simulink model "Control_v4_desat0"  (R2020b)
settings: Solver=FixedStepAuto  StartTime=0.0  StopTime=t_sim  FixedStep=TimeStep  RelTol=1e-3
values from neighbouring files (symbols this model uses):
  date_IGRF = [date.year,date.month,date.day]    [main_SCA_v3.m]
  MODE = 2    [main_SCA_alt.m]    (also in main_SCA_v3.m)
  nmax = 2    [main_SCA.m]    (also in main_SCA_alt.m; main_SCA_v3.m)
  Use_IGRF = 0    [main_SCA.m]    (also in main_SCA_alt.m; main_SCA_v3.m)
undefined symbols (not defined in the file or in its folder): att, date, deg, DipoleMod, DiscIntNeverNeededParam, IonSataero, km, orbit, rad, s, sat
libraries: vrlib x16, aerolibconvert2 x13, aerolibutil x13, sharedtransform x11, dspmathops x10, simulink x5, sharedutil x3, simulink_extras x2, dspstat3 x1, aerolibatmos2 x1, aerolibobsolete x1, aerolibcelestial x1
(part 2 of 3)

== system Control_v4_desat0/Physical Model/Magnetorquer physics ==
  note: On pourrait aussi changer les blocs
      | magnétocoupleurs pour sortir les intensités
  Mag vector command : Inport
  B_IGRF_body (vecteur) : Inport  Port=2
  Add1 : Sum  Inputs=+++
  Cross Product : vrlib/Utilities/Cross Product
  Demux : Demux  Outputs=3
  Magnétocoupleur 1 : Subsystem
  Magnétocoupleur 2 : Subsystem
  Magnétocoupleur 3 : Subsystem
  Couple (vect) : Outport  PortDimensions=3  VectorParamsAs1DForOutWhenUnconnected=off
  Real mag moments vector : Outport  Port=2  VectorParamsAs1DForOutWhenUnconnected=off
  wires:
  Add1/1 -> Real mag moments vector/1, Cross Product/1  "M_real"
  Demux/1 -> Magnétocoupleur 1/1(m_in (scalar))
  Demux/2 -> Magnétocoupleur 2/1(m_in (scalar))
  Demux/3 -> Magnétocoupleur 3/1(m_in (scalar))
  Mag vector command/1 -> Demux/1  "m_c"
  Magnétocoupleur 2/1(m_out (vect)) -> Add1/2
  Magnétocoupleur 1/1(m_out (vect)) -> Add1/1
  Magnétocoupleur 3/1(m_out (vect)) -> Add1/3
  Cross Product/1 -> Couple (vect)/1  "T_body"
  B_IGRF_body (vecteur)/1 -> Cross Product/2

== system Control_v4_desat0/Physical Model/Thruster ==
  On/Off (Boolean) : Inport  OutDataTypeStr=boolean
  Constant : Constant  Value=0
  Cross Product : vrlib/Utilities/Cross Product
  If : If  IfExpression=u1
  If Action Subsystem : Subsystem  TreatAsAtomicUnit=on
  If Action Subsystem1 : Subsystem  TreatAsAtomicUnit=on
  Merge : Merge
  Product : Product
  Sum : Sum  Inputs=|+-
  Thruster Force : Constant  Value=sat.thruster.force
  unit vector of thrust : Constant  Value=sat.thruster.dir
  vector G-Thrust point : Constant  Value=sat.thruster.point
  vector G-Thrust point1 : Constant  Value=sat.CoG
  Force (G_sat) : Outport  VectorParamsAs1DForOutWhenUnconnected=off
  Moment (G_sat) : Outport  Port=2  VectorParamsAs1DForOutWhenUnconnected=off
  wires:
  Product/1 -> Force (G_sat)/1, Cross Product/2
  Sum/1 -> Cross Product/1
  unit vector of thrust/1 -> Product/1
  Cross Product/1 -> Moment (G_sat)/1
  Thruster Force/1 -> If Action Subsystem/1(In1)
  On/Off (Boolean)/1 -> If/1
  If/1 -> If Action Subsystem/Action
  If/2 -> If Action Subsystem1/Action
  If Action Subsystem1/1(Out1) -> Merge/2
  If Action Subsystem/1(Out1) -> Merge/1
  Merge/1 -> Product/2
  Constant/1 -> If Action Subsystem1/1(In1)
  vector G-Thrust point/1 -> Sum/1
  vector G-Thrust point1/1 -> Sum/2

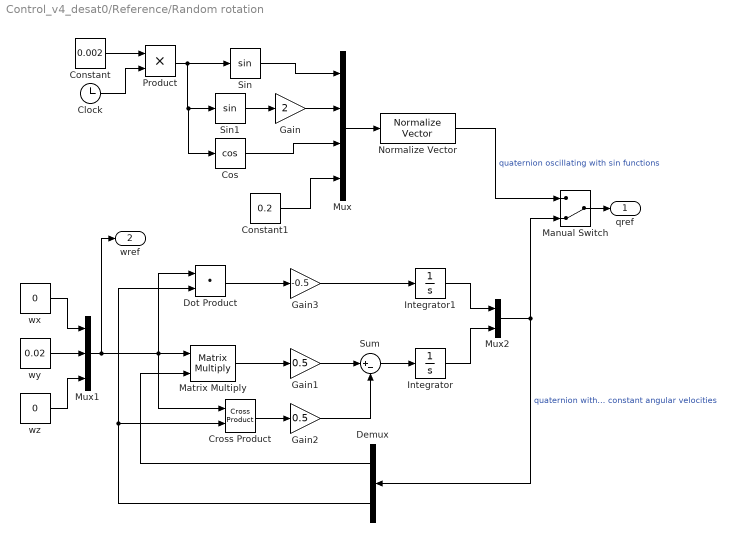
== system Control_v4_desat0/Reference/Random rotation ==
  Clock : Clock
      settings: Decimation=TimeStep
  Constant : Constant  Value=0.002
  Constant1 : Constant  Value=0.2
  Cos : Trigonometry  Operator=cos
  Cross Product : vrlib/Utilities/Cross Product
  Demux : Demux  Outputs=[1;3]
  Dot Product : DotProduct  InputSameDT=on  OutDataTypeStr=Inherit: Inherit via internal rule
  Gain : Gain  Gain=2
  Gain1 : Gain  Gain=0.5
  Gain2 : Gain  Gain=0.5
  Gain3 : Gain  Gain=-0.5
  Integrator : Integrator  InitialCondition=[0;0;0]
  Integrator1 : Integrator  InitialCondition=1
  Manual Switch : ManualSwitch  CurrentSetting=0
  Matrix Multiply : Product  Multiplication=Matrix(*)
  Mux : Mux
  Mux1 : Mux  Inputs=3
  Mux2 : Mux  Inputs=[1;3]
  Normalize Vector : vrlib/Utilities/Normalize Vector  maxzero=0
  Product : Product
  Sin : Trigonometry
  Sin1 : Trigonometry
  Sum : Sum  Inputs=|+-
  wx : Constant  Value=0
  wy : Constant  Value=0.02
  wz : Constant  Value=0
  qref : Outport
  wref : Outport  Port=2
  wires:
  Mux/1 -> Normalize Vector/1
  Normalize Vector/1 -> Manual Switch/1  "quaternion oscillating with sin functions"
  Constant/1 -> Product/1
  Clock/1 -> Product/2
  Product/1 -> Cos/1, Sin1/1, Sin/1
  Sin/1 -> Mux/1
  Sin1/1 -> Gain/1
  Gain/1 -> Mux/2
  Cos/1 -> Mux/3
  Constant1/1 -> Mux/4
  Manual Switch/1 -> qref/1
  wx/1 -> Mux1/1
  wy/1 -> Mux1/2
  wz/1 -> Mux1/3
  Mux1/1 -> wref/1, Dot Product/1, Cross Product/1, Matrix Multiply/1
  Matrix Multiply/1 -> Gain1/1
  Gain1/1 -> Sum/1
  Sum/1 -> Integrator/1
  Integrator/1 -> Mux2/2
  Mux2/1 -> Demux/1, Manual Switch/2  "quaternion with constant angular velocities"
  Demux/1 -> Matrix Multiply/2
  Cross Product/1 -> Gain2/1
  Gain2/1 -> Sum/2
  Dot Product/1 -> Gain3/1
  Gain3/1 -> Integrator1/1
  Integrator1/1 -> Mux2/1
  Demux/2 -> Cross Product/2, Dot Product/2

== system Control_v4_desat0/Reference/Switch Case Action Subsystem ==
  Q_orbit : Inport
  W_orbit1 : Inport  Port=2
  Action Port : ActionPort  ActionPortLabel=default:
  Out1 : Outport  VectorParamsAs1DForOutWhenUnconnected=off
  Out3 : Outport  Port=2  VectorParamsAs1DForOutWhenUnconnected=off
  wires:
  Q_orbit/1 -> Out1/1
  W_orbit1/1 -> Out3/1

== system Control_v4_desat0/Reference/Switch Case Action Subsystem1 ==
  Q_retro : Inport
  W_retro : Inport  Port=2
  Action Port : ActionPort  ActionPortLabel=case [ 5 ]:
  Out1 : Outport  VectorParamsAs1DForOutWhenUnconnected=off
  Out3 : Outport  Port=2  VectorParamsAs1DForOutWhenUnconnected=off
  wires:
  Q_retro/1 -> Out1/1
  W_retro/1 -> Out3/1

== system Control_v4_desat0/Reference/Switch Case Action Subsystem2 ==
  note: q from I to O + rotation
  Q_drag : Inport
  W_drag : Inport  Port=2
  Action Port : ActionPort  ActionPortLabel=case [ 4 ]:
  Out1 : Outport  VectorParamsAs1DForOutWhenUnconnected=off
  W : Outport  Port=2
  wires:
  Q_drag/1 -> Out1/1
  W_drag/1 -> W/1

== system Control_v4_desat0/Reference/Switch Case Action Subsystem3 ==
  Q_sun_sun : Inport
  W_sun_sun : Inport  Port=2
  Action Port : ActionPort  ActionPortLabel=case [ 3 ]:
  Out1 : Outport  VectorParamsAs1DForOutWhenUnconnected=off
  Out3 : Outport  Port=2  VectorParamsAs1DForOutWhenUnconnected=off
  wires:
  Q_sun_sun/1 -> Out1/1
  W_sun_sun/1 -> Out3/1

== system Control_v4_desat0/Reference/Switch Case Action Subsystem4 ==
  Q_sun_aero : Inport
  W_sun_aero : Inport  Port=2
  Action Port : ActionPort  ActionPortLabel=case [ 2 ]:
  Out1 : Outport  VectorParamsAs1DForOutWhenUnconnected=off
  Out3 : Outport  Port=2  VectorParamsAs1DForOutWhenUnconnected=off
  wires:
  Q_sun_aero/1 -> Out1/1
  W_sun_aero/1 -> Out3/1

== system Control_v4_desat0/Reference/Switch Case Action Subsystem5 ==
  In1 : Inport
  W_orbit : Inport  Port=2
  Action Port : ActionPort  ActionPortLabel=case [ 1 ]:
  Out1 : Outport  VectorParamsAs1DForOutWhenUnconnected=off
  Out3 : Outport  Port=2  VectorParamsAs1DForOutWhenUnconnected=off
  wires:
  In1/1 -> Out1/1
  W_orbit/1 -> Out3/1

== system Control_v4_desat0/Reference/Switch Case Action Subsystem6 ==
  In1 : Inport
  In2 : Inport  Port=2
  Action Port : ActionPort  ActionPortLabel=case [ 7 ]:
  Derivative : Derivative
  Matrix Multiply : Product  Multiplication=Matrix(*)
  Quaternions to Direction Cosine Matrix : sharedtransform/Quaternions to  Direction Cosine Matrix  aMode=aMode
      settings: SourceProductBaseCode=AE,PW,MT,UV,VE,VP
  Transpose : Math  Operator=transpose  SaturateOnIntegerOverflow=on
  Transpose1 : Math  Operator=transpose  SaturateOnIntegerOverflow=on
  gets vector from Skew Matrix : MATLABFcn  MATLABFcn=vec_from_skew
  Out1 : Outport  VectorParamsAs1DForOutWhenUnconnected=off
  W_custom : Outport  Port=2
  wires:
  In1/1 -> Out1/1
  In2/1 -> Quaternions to Direction Cosine Matrix/1
  Quaternions to Direction Cosine Matrix/1 -> Transpose1/1
  Matrix Multiply/1 -> gets vector from Skew Matrix/1
  Transpose/1 -> Derivative/1
  gets vector from Skew Matrix/1 -> W_custom/1
  Derivative/1 -> Matrix Multiply/1
  Transpose1/1 -> Transpose/1, Matrix Multiply/2

== system Control_v4_desat0/Reference/Switch Case Action Subsystem7 ==
  In1 : Inport
  In2 : Inport  Port=2
  Action Port : ActionPort  ActionPortLabel=case [ 6 ]:
  Out1 : Outport  VectorParamsAs1DForOutWhenUnconnected=off
  Out2 : Outport  Port=2  VectorParamsAs1DForOutWhenUnconnected=off
  wires:
  In1/1 -> Out1/1
  In2/1 -> Out2/1

== system Control_v4_desat0/Reference/q_drag ==
  note: DCM from Drag to Inertial
  note: q from D to I
  note: q from I to D
  note: To get angular velocity from Rotation matrix:
      | https://en.wikipedia.org/wiki/Angular_velocity#Angular_velocity_tensor
      | W= dA/dt * A'
      | $W=\frac{dA}{dt} {\dot} A'=\frac{dA}{dt} {\dot} A^{T}$
  <XYZ_ECI> : Inport
  <VxVyVz_ECI> : Inport  Port=2
  3x3 Cross Product : sharedutil/3x3 Cross Product  aMode=aMode
      settings: SourceProductBaseCode=AE,PW,MT,UV,VE,VP
  Derivative : Derivative
  Direction Cosine Matrix to Quaternions : sharedtransform/Direction Cosine Matrix  to Quaternions  aMode=0  action=None  tolerance=eps(2)
      settings: SourceProductBaseCode=AE,PW,MT,UV,VE,VP
  Gain : Gain
  Gain1 : Gain
  Matrix Multiply : Product  Multiplication=Matrix(*)
  Normalization : dspmathops/Normalization  NormType=2-norm  Bias=1e-10  NormOver=Each column  Dimension=1  roundingMode=Floor  overflowMode=off  accumDataTypeStr=Inherit: Same as product output  accumLastDataTypeStr=Inherit: Same as product output  outputDataTypeStr=Inherit: Same as product output  outputMin=[]  outputMax=[]  outputLastDataTypeStr=Inherit: Same as product output
  Normalization1 : dspmathops/Normalization  NormType=2-norm  Bias=1e-10  NormOver=Each column  Dimension=1  roundingMode=Floor  overflowMode=off  accumDataTypeStr=Inherit: Same as product output  accumLastDataTypeStr=Inherit: Same as product output  outputDataTypeStr=Inherit: Same as product output  outputMin=[]  outputMax=[]  outputLastDataTypeStr=Inherit: Same as product output
  Quaternion Inverse : aerolibutil/Quaternion Inverse
  Reshape : Reshape  OutputDimensionality=Column vector (2-D)
  Reshape1 : Reshape  OutputDimensionality=Column vector (2-D)
  Reshape2 : Reshape  OutputDimensionality=Column vector (2-D)
  Reshape3 : Reshape  OutputDimensionality=Customize  OutputDimensions=[3,3]
  Transpose : Math  Operator=transpose  SaturateOnIntegerOverflow=on
  Vector Concatenate : Concatenate  NumInputs=3  Mode=Multidimensional array  ConcatenateDimension=2
  gets vector from Skew Matrix : MATLABFcn  MATLABFcn=vec_from_skew
  Q_drag : Outport  VectorParamsAs1DForOutWhenUnconnected=off
  W_drag : Outport  Port=2
  wires:
  Normalization/1 -> Reshape/1
  Normalization1/1 -> Reshape1/1
  <VxVyVz_ECI>/1 -> Normalization1/1
  Reshape1/1 -> Vector Concatenate/3, 3x3 Cross Product/1
  <XYZ_ECI>/1 -> Normalization/1
  Reshape/1 -> Gain/1
  Gain/1 -> Vector Concatenate/1, 3x3 Cross Product/2
  Direction Cosine Matrix to Quaternions/1 -> Quaternion Inverse/1
  3x3 Cross Product/1 -> Gain1/1
  Gain1/1 -> Reshape2/1
  Quaternion Inverse/1 -> Q_drag/1
  Vector Concatenate/1 -> Reshape3/1, Direction Cosine Matrix to Quaternions/1
  gets vector from Skew Matrix/1 -> W_drag/1
  Matrix Multiply/1 -> gets vector from Skew Matrix/1
  Transpose/1 -> Derivative/1
  Derivative/1 -> Matrix Multiply/1
  Reshape2/1 -> Vector Concatenate/2
  Reshape3/1 -> Matrix Multiply/2, Transpose/1

== system Control_v4_desat0/Reference/q_orbital ==
  note: DCM from Orbital to Inertial
  note: q from O to I
  note: q from I to O
  note: To get angular velocity from Rotation matrix:
      | https://en.wikipedia.org/wiki/Angular_velocity#Angular_velocity_tensor
      | W= dA/dt * A'
      | $W=\frac{dA}{dt} {\dot} A'=\frac{dA}{dt} {\dot} A^{T}$
  <XYZ_ECI> : Inport
  <VxVyVz_ECI> : Inport  Port=2
  3x3 Cross Product : sharedutil/3x3 Cross Product  aMode=aMode
      settings: SourceProductBaseCode=AE,PW,MT,UV,VE,VP
  Derivative : Derivative
  Direction Cosine Matrix to Quaternions : sharedtransform/Direction Cosine Matrix  to Quaternions  aMode=0  action=None  tolerance=eps(2)
      settings: SourceProductBaseCode=AE,PW,MT,UV,VE,VP
  Gain : Gain
  Gain1 : Gain  Gain=-1
  Matrix Multiply : Product  Multiplication=Matrix(*)
  Normalization : dspmathops/Normalization  NormType=2-norm  Bias=1e-10  NormOver=Each column  Dimension=1  roundingMode=Floor  overflowMode=off  accumDataTypeStr=Inherit: Same as product output  accumLastDataTypeStr=Inherit: Same as product output  outputDataTypeStr=Inherit: Same as product output  outputMin=[]  outputMax=[]  outputLastDataTypeStr=Inherit: Same as product output
  Normalization1 : dspmathops/Normalization  NormType=2-norm  Bias=1e-10  NormOver=Each column  Dimension=1  roundingMode=Floor  overflowMode=off  accumDataTypeStr=Inherit: Same as product output  accumLastDataTypeStr=Inherit: Same as product output  outputDataTypeStr=Inherit: Same as product output  outputMin=[]  outputMax=[]  outputLastDataTypeStr=Inherit: Same as product output
  Quaternion Inverse : aerolibutil/Quaternion Inverse
  Reshape : Reshape  OutputDimensionality=Column vector (2-D)
  Reshape1 : Reshape  OutputDimensionality=Column vector (2-D)
  Reshape2 : Reshape  OutputDimensionality=Column vector (2-D)
  Reshape3 : Reshape  OutputDimensionality=Customize  OutputDimensions=[3,3]
  Transpose : Math  Operator=transpose  SaturateOnIntegerOverflow=on
  Vector Concatenate : Concatenate  NumInputs=3  Mode=Multidimensional array  ConcatenateDimension=2
  gets vector from Skew Matrix : MATLABFcn  MATLABFcn=vec_from_skew
  Q_orbit : Outport  VectorParamsAs1DForOutWhenUnconnected=off
  W_orbit : Outport  Port=2
  wires:
  Normalization/1 -> Reshape/1
  Normalization1/1 -> Reshape1/1
  <VxVyVz_ECI>/1 -> Normalization1/1
  Reshape1/1 -> 3x3 Cross Product/1, Vector Concatenate/1
  <XYZ_ECI>/1 -> Normalization/1
  Reshape/1 -> Gain/1
  Gain/1 -> 3x3 Cross Product/2, Vector Concatenate/3
  Direction Cosine Matrix to Quaternions/1 -> Quaternion Inverse/1
  3x3 Cross Product/1 -> Gain1/1
  Gain1/1 -> Reshape2/1
  Quaternion Inverse/1 -> Q_orbit/1
  Vector Concatenate/1 -> Reshape3/1, Direction Cosine Matrix to Quaternions/1
  gets vector from Skew Matrix/1 -> W_orbit/1
  Matrix Multiply/1 -> gets vector from Skew Matrix/1
  Transpose/1 -> Derivative/1
  Derivative/1 -> Matrix Multiply/1
  Reshape2/1 -> Vector Concatenate/2
  Reshape3/1 -> Matrix Multiply/2, Transpose/1

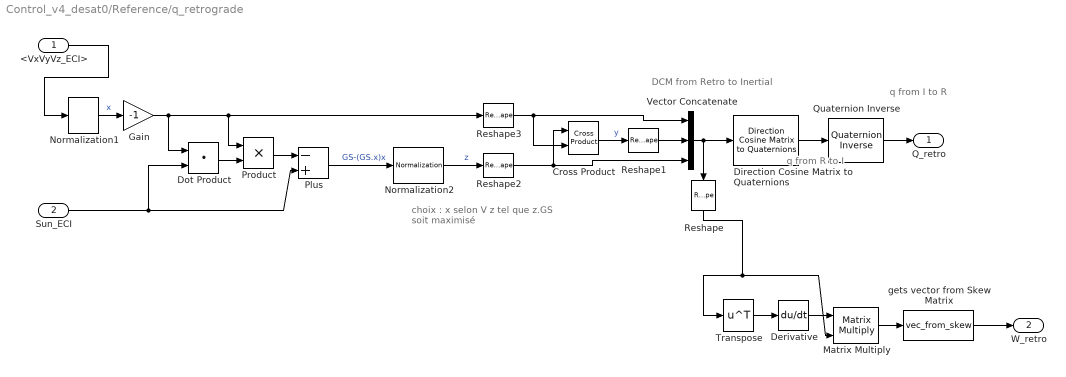
== system Control_v4_desat0/Reference/q_retrograde ==
  note: q from I to R
  note: q from R to I
  note: DCM from Retro to Inertial
  note: choix :
      | x selon V
      | z tel que z.GS soit maximisé
  <VxVyVz_ECI> : Inport
  Sun_ECI : Inport  Port=2
  Cross Product : vrlib/Utilities/Cross Product
  Derivative : Derivative
  Direction Cosine Matrix to Quaternions : sharedtransform/Direction Cosine Matrix  to Quaternions  aMode=0  action=None  tolerance=eps(2)
      settings: SourceProductBaseCode=AE,PW,MT,UV,VE,VP
  Dot Product : DotProduct  InputSameDT=on  OutDataTypeStr=Inherit: Inherit via internal rule
  Gain : Gain  Gain=-1
  Matrix Multiply : Product  Multiplication=Matrix(*)
  Normalization1 : dspmathops/Normalization  NormType=2-norm  Bias=1e-10  NormOver=Each column  Dimension=1  roundingMode=Floor  overflowMode=off  accumDataTypeStr=Inherit: Same as product output  accumLastDataTypeStr=Inherit: Same as product output  outputDataTypeStr=Inherit: Same as product output  outputMin=[]  outputMax=[]  outputLastDataTypeStr=Inherit: Same as product output
  Normalization2 : dspmathops/Normalization  NormType=2-norm  Bias=1e-10  NormOver=Each column  Dimension=1  roundingMode=Floor  overflowMode=off  accumDataTypeStr=Inherit: Same as product output  accumLastDataTypeStr=Inherit: Same as product output  outputDataTypeStr=Inherit: Same as product output  outputMin=[]  outputMax=[]  outputLastDataTypeStr=Inherit: Same as product output
  Plus : Sum  Inputs=-+
  Product : Product
  Quaternion Inverse : aerolibutil/Quaternion Inverse
  Reshape : Reshape  OutputDimensionality=Customize  OutputDimensions=[3,3]
  Reshape1 : Reshape  OutputDimensionality=Column vector (2-D)
  Reshape2 : Reshape  OutputDimensionality=Column vector (2-D)
  Reshape3 : Reshape  OutputDimensionality=Column vector (2-D)
  Transpose : Math  Operator=transpose  SaturateOnIntegerOverflow=on
  Vector Concatenate : Concatenate  NumInputs=3  Mode=Multidimensional array  ConcatenateDimension=2
  gets vector from Skew Matrix : MATLABFcn  MATLABFcn=vec_from_skew
  Q_retro : Outport  VectorParamsAs1DForOutWhenUnconnected=off
  W_retro : Outport  Port=2
  wires:
  Quaternion Inverse/1 -> Q_retro/1
  Reshape2/1 -> Vector Concatenate/3, Cross Product/1
  Reshape3/1 -> Vector Concatenate/1, Cross Product/2
  Product/1 -> Plus/1
  Dot Product/1 -> Product/2
  Cross Product/1 -> Reshape1/1  "y"
  Normalization2/1 -> Reshape2/1  "z"
  Plus/1 -> Normalization2/1  "GS-(GS.x)x"
  Sun_ECI/1 -> Dot Product/2, Plus/2
  Direction Cosine Matrix to Quaternions/1 -> Quaternion Inverse/1
  Normalization1/1 -> Gain/1  "x"
  <VxVyVz_ECI>/1 -> Normalization1/1
  Reshape1/1 -> Vector Concatenate/2
  Gain/1 -> Dot Product/1, Product/1, Reshape3/1
  Vector Concatenate/1 -> Direction Cosine Matrix to Quaternions/1, Reshape/1
  gets vector from Skew Matrix/1 -> W_retro/1
  Matrix Multiply/1 -> gets vector from Skew Matrix/1
  Derivative/1 -> Matrix Multiply/1
  Transpose/1 -> Derivative/1
  Reshape/1 -> Transpose/1, Matrix Multiply/2

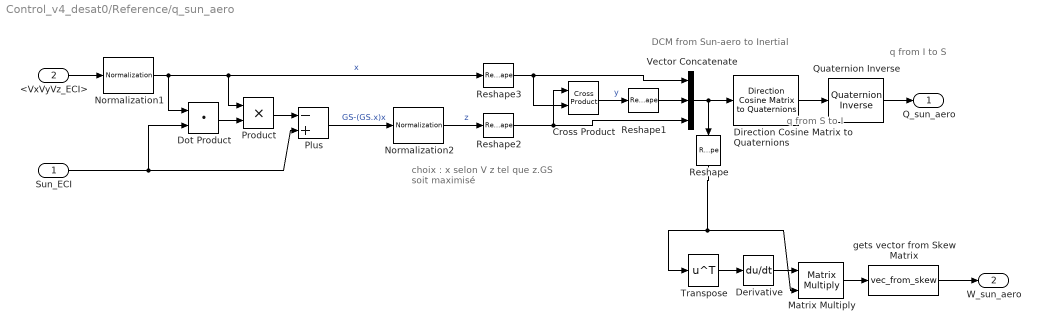
== system Control_v4_desat0/Reference/q_sun_aero ==
  note: q from I to S
  note: q from S to I
  note: DCM from Sun-aero to Inertial
  note: choix :
      | x selon V
      | z tel que z.GS soit maximisé
  Sun_ECI : Inport
  <VxVyVz_ECI> : Inport  Port=2
  Cross Product : vrlib/Utilities/Cross Product
  Derivative : Derivative
  Direction Cosine Matrix to Quaternions : sharedtransform/Direction Cosine Matrix  to Quaternions  aMode=0  action=None  tolerance=eps(2)
      settings: SourceProductBaseCode=AE,PW,MT,UV,VE,VP
  Dot Product : DotProduct  InputSameDT=on  OutDataTypeStr=Inherit: Inherit via internal rule
  Matrix Multiply : Product  Multiplication=Matrix(*)
  Normalization1 : dspmathops/Normalization  NormType=2-norm  Bias=1e-10  NormOver=Each column  Dimension=1  roundingMode=Floor  overflowMode=off  accumDataTypeStr=Inherit: Same as product output  accumLastDataTypeStr=Inherit: Same as product output  outputDataTypeStr=Inherit: Same as product output  outputMin=[]  outputMax=[]  outputLastDataTypeStr=Inherit: Same as product output
  Normalization2 : dspmathops/Normalization  NormType=2-norm  Bias=1e-10  NormOver=Each column  Dimension=1  roundingMode=Floor  overflowMode=off  accumDataTypeStr=Inherit: Same as product output  accumLastDataTypeStr=Inherit: Same as product output  outputDataTypeStr=Inherit: Same as product output  outputMin=[]  outputMax=[]  outputLastDataTypeStr=Inherit: Same as product output
  Plus : Sum  Inputs=-+
  Product : Product
  Quaternion Inverse : aerolibutil/Quaternion Inverse
  Reshape : Reshape  OutputDimensionality=Customize  OutputDimensions=[3,3]
  Reshape1 : Reshape  OutputDimensionality=Column vector (2-D)
  Reshape2 : Reshape  OutputDimensionality=Column vector (2-D)
  Reshape3 : Reshape  OutputDimensionality=Column vector (2-D)
  Transpose : Math  Operator=transpose  SaturateOnIntegerOverflow=on
  Vector Concatenate : Concatenate  NumInputs=3  Mode=Multidimensional array  ConcatenateDimension=2
  gets vector from Skew Matrix : MATLABFcn  MATLABFcn=vec_from_skew
  Q_sun_aero : Outport  VectorParamsAs1DForOutWhenUnconnected=off
  W_sun_aero : Outport  Port=2
  wires:
  Quaternion Inverse/1 -> Q_sun_aero/1
  Reshape2/1 -> Vector Concatenate/3, Cross Product/1
  Reshape3/1 -> Vector Concatenate/1, Cross Product/2
  Product/1 -> Plus/1
  Dot Product/1 -> Product/2
  Cross Product/1 -> Reshape1/1  "y"
  Normalization2/1 -> Reshape2/1  "z"
  Plus/1 -> Normalization2/1  "GS-(GS.x)x"
  Sun_ECI/1 -> Dot Product/2, Plus/2
  Direction Cosine Matrix to Quaternions/1 -> Quaternion Inverse/1
  Normalization1/1 -> Dot Product/1, Product/1, Reshape3/1  "x"
  <VxVyVz_ECI>/1 -> Normalization1/1
  Reshape1/1 -> Vector Concatenate/2
  Transpose/1 -> Derivative/1
  Matrix Multiply/1 -> gets vector from Skew Matrix/1
  Derivative/1 -> Matrix Multiply/1
  Vector Concatenate/1 -> Direction Cosine Matrix to Quaternions/1, Reshape/1
  gets vector from Skew Matrix/1 -> W_sun_aero/1
  Reshape/1 -> Transpose/1, Matrix Multiply/2

== system Control_v4_desat0/Reference/q_sun_sun ==
  note: Choix:
      | z selon GS
      | x tel que x.V soit maximisé
  note: DCM from Sun-sun to Inertial
  note: q from I to SS
  note: q from SS to I
  <VxVyVz_ECI> : Inport
  Sun_ECI : Inport  Port=2
  Cross Product1 : vrlib/Utilities/Cross Product
  Derivative : Derivative
  Direction Cosine Matrix to Quaternions1 : sharedtransform/Direction Cosine Matrix  to Quaternions  aMode=0  action=None  tolerance=eps(2)
      settings: SourceProductBaseCode=AE,PW,MT,UV,VE,VP
  Dot Product1 : DotProduct  InputSameDT=on  OutDataTypeStr=Inherit: Inherit via internal rule
  Matrix Multiply : Product  Multiplication=Matrix(*)
  Normalization3 : dspmathops/Normalization  NormType=2-norm  Bias=1e-10  NormOver=Each column  Dimension=1  roundingMode=Floor  overflowMode=off  accumDataTypeStr=Inherit: Same as product output  accumLastDataTypeStr=Inherit: Same as product output  outputDataTypeStr=Inherit: Same as product output  outputMin=[]  outputMax=[]  outputLastDataTypeStr=Inherit: Same as product output
  Normalization4 : dspmathops/Normalization  NormType=2-norm  Bias=1e-10  NormOver=Each column  Dimension=1  roundingMode=Floor  overflowMode=off  accumDataTypeStr=Inherit: Same as product output  accumLastDataTypeStr=Inherit: Same as product output  outputDataTypeStr=Inherit: Same as product output  outputMin=[]  outputMax=[]  outputLastDataTypeStr=Inherit: Same as product output
  Plus1 : Sum  Inputs=-+
  Product1 : Product
  Quaternion Inverse1 : aerolibutil/Quaternion Inverse
  Reshape : Reshape  OutputDimensionality=Customize  OutputDimensions=[3,3]
  Reshape4 : Reshape  OutputDimensionality=Column vector (2-D)
  Reshape5 : Reshape  OutputDimensionality=Column vector (2-D)
  Reshape6 : Reshape  OutputDimensionality=Column vector (2-D)
  Transpose : Math  Operator=transpose  SaturateOnIntegerOverflow=on
  Vector Concatenate1 : Concatenate  NumInputs=3  Mode=Multidimensional array  ConcatenateDimension=2
  gets vector from Skew Matrix : MATLABFcn  MATLABFcn=vec_from_skew
  Q_sun_sun : Outport  VectorParamsAs1DForOutWhenUnconnected=off
  W_sun_sun : Outport  Port=2
  wires:
  Direction Cosine Matrix to Quaternions1/1 -> Quaternion Inverse1/1
  Reshape4/1 -> Vector Concatenate1/2
  Dot Product1/1 -> Product1/1
  Sun_ECI/1 -> Normalization3/1
  Quaternion Inverse1/1 -> Q_sun_sun/1
  <VxVyVz_ECI>/1 -> Dot Product1/1, Plus1/1
  Plus1/1 -> Normalization4/1  "V-(V.z)z"
  Reshape6/1 -> Cross Product1/1, Vector Concatenate1/3
  Normalization3/1 -> Dot Product1/2, Product1/2, Reshape6/1  "z"
  Reshape5/1 -> Cross Product1/2, Vector Concatenate1/1
  Cross Product1/1 -> Reshape4/1  "y"
  Normalization4/1 -> Reshape5/1  "x"
  Product1/1 -> Plus1/2
  Reshape/1 -> Matrix Multiply/2, Transpose/1
  Derivative/1 -> Matrix Multiply/1
  Transpose/1 -> Derivative/1
  Matrix Multiply/1 -> gets vector from Skew Matrix/1
  gets vector from Skew Matrix/1 -> W_sun_sun/1
  Vector Concatenate1/1 -> Direction Cosine Matrix to Quaternions1/1, Reshape/1

== system Control_v4_desat0/Attitude Controller/Magnetorquer Magnetic Momend Command/Switch Case Action Subsystem3 ==
  In1 : Inport
  Action Port : ActionPort  ActionPortLabel=if(u1 > 0)
  Out1 : Outport  VectorParamsAs1DForOutWhenUnconnected=off
  wires:
  In1/1 -> Out1/1

== system Control_v4_desat0/Attitude Controller/Magnetorquer Magnetic Momend Command/Switch Case Action Subsystem4 ==
  In1 : Inport
  Action Port : ActionPort  ActionPortLabel=else
  Out1 : Outport  VectorParamsAs1DForOutWhenUnconnected=off
  wires:
  In1/1 -> Out1/1

== system Control_v4_desat0/Attitude Controller/PID (nominal command)/Command Magnetic moments computation ==
  note: Moment magnétique de commande m_c :
      |
      | $m_c = \frac{1}{B²}\vec{B} \wedge\vec{T_C}$
      | Avec Tp couple projeté dans le plan orthogonal à B ( On aura ainsi un couple effectif égal à la projection du couple de consigne idéal projeté dans le plan orthogonal au champ local )
      | $T_{eff}=\vec{T_{C}}-\frac{1}{B²}(\vec{T_{C}}\cdot\vec{B})\vec{B}$
      | Avec Tc couple projeté dans le plan orthogonal à B
      |
      | $\vec{T_c} =k_{mag} \vec{\omega_{rw}}$
      |
      | Moment magnétique de commande m_c :
      | $\vec{m_c} = \frac{k_{mag}}{B²}\vec{B} \wedge\vec{\omega_{RW}}$
  Command (vect) : Inport  OutDataTypeStr=double
  B_IGRF_body (vect) : Inport  Port=2  OutDataTypeStr=double
  h1 (vect) : Inport  Port=3
  h2 (vect) : Inport  Port=4
  h3 (vect) : Inport  Port=5
  Cross Product : vrlib/Utilities/Cross Product
  Dot Product : DotProduct  InputSameDT=on  OutDataTypeStr=Inherit: Inherit via internal rule
  Global magnetic moment computation : Subsystem
  Mux : Mux  Inputs=3
  Product1 : Product  Inputs=*/
  Reshape : Reshape  OutputDimensionality=Column vector (2-D)
  Reshape1 : Reshape  OutputDimensionality=Column vector (2-D)
  Mag vector command : Outport  VectorParamsAs1DForOutWhenUnconnected=off
  wires:
  B_IGRF_body (vect)/1 -> Reshape1/1  "B_Body"
  Command (vect)/1 -> Reshape/1  "T_Body"
  h1 (vect)/1 -> Global magnetic moment computation/2(In2)
  h2 (vect)/1 -> Global magnetic moment computation/3(In3)
  h3 (vect)/1 -> Global magnetic moment computation/4(In4)
  Global magnetic moment computation/2(magnetic moment 2 (scalar)) -> Mux/2  "magnetic moment 2"
  Global magnetic moment computation/3(magnetic moment 3 (scalar)) -> Mux/3  "magnetic moment 3"
  Global magnetic moment computation/1(magnetic moment 1 (scalar)) -> Mux/1  "magnetic moment 1"
  Mux/1 -> Mag vector command/1
  Reshape1/1 -> Cross Product/2, Dot Product/2, Dot Product/1
  Cross Product/1 -> Product1/1
  Product1/1 -> Global magnetic moment computation/1(In1)  "m_c"
  Dot Product/1 -> Product1/2  "B^2"
  Reshape/1 -> Cross Product/1  "Tc"

== system Control_v4_desat0/Attitude Controller/PID (nominal command)/Extract Vect ==
  Qr : Inport
  Demux : Demux
  Mux1 : Mux  Inputs=3
  Product : Product
  Reshape : Reshape  OutputDimensionality=Column vector (2-D)
  Sign : Signum
  Qvect : Outport  VectorParamsAs1DForOutWhenUnconnected=off
  wires:
  Demux/2 -> Mux1/1
  Demux/4 -> Mux1/3
  Demux/3 -> Mux1/2
  Demux/1 -> Sign/1
  Qr/1 -> Demux/1
  Mux1/1 -> Product/2
  Product/1 -> Reshape/1
  Sign/1 -> Product/1
  Reshape/1 -> Qvect/1

== system Control_v4_desat0/Attitude Controller/PID (nominal command)/If Action Subsystem ==
  In1 : Inport
  Action Port : ActionPort  ActionPortLabel=else
  Out1 : Outport  VectorParamsAs1DForOutWhenUnconnected=off
  wires:
  In1/1 -> Out1/1

== system Control_v4_desat0/Attitude Controller/PID (nominal command)/If Action Subsystem1 ==
  In1 : Inport
  Action Port : ActionPort  ActionPortLabel=if(u1 > 0)
  Out1 : Outport  VectorParamsAs1DForOutWhenUnconnected=off
  wires:
  In1/1 -> Out1/1

== system Control_v4_desat0/Attitude Controller/PID (nominal command)/If Action Subsystem2 ==
  In1 : Inport
  Action Port : ActionPort  ActionPortLabel=if(u1 > 0.0068)
  Out1 : Outport  VectorParamsAs1DForOutWhenUnconnected=off
  wires:
  In1/1 -> Out1/1

== system Control_v4_desat0/Attitude Controller/PID (nominal command)/If Action Subsystem3 ==
  In1 : Inport
  Action Port : ActionPort  ActionPortLabel=else
  Out1 : Outport  VectorParamsAs1DForOutWhenUnconnected=off
  wires:
  In1/1 -> Out1/1

== system Control_v4_desat0/Attitude Controller/PID (nominal command)/If Action Subsystem4 ==
  In1 : Inport
  Action Port : ActionPort  ActionPortLabel=else
  Out1 : Outport
  wires:
  In1/1 -> Out1/1

== system Control_v4_desat0/Attitude Controller/PID (nominal command)/If Action Subsystem6 ==
  In1 : Inport
  Action Port : ActionPort  ActionPortLabel=if(u1 ~= 0)
  Gain1 : Gain  Gain=20
  Out1 : Outport
  wires:
  In1/1 -> Gain1/1
  Gain1/1 -> Out1/1

== system Control_v4_desat0/Attitude Controller/PID (nominal command)/RW1 ==
  note: Actuator power models:
      | https://digitalcommons.usu.edu/cgi/viewcontent.cgi?article=1080&context=smallsat
      | $P_{rw}=1000T+4.5h^{0.47}$
  note: Entrées:
      | - Moment de commande (déjà projeté sur l'axe de la roue...)
      | Sorties:
      | - Omega de commande à appliquer
  Mc (scalar) : Inport
  Discrete-Time Integrator : DiscreteIntegrator  IntegratorMethod=Integration: Trapezoidal  SampleTime=-1  ICPrevOutput=DiscIntNeverNeededParam  ICPrevScaledInput=DiscIntNeverNeededParam
  Divide : Product  Inputs=*/
  Saturation_speed : Saturate  UpperLimit=sat.wheel.max_speed  LowerLimit=- sat.wheel.max_speed
  Subsystem : Subsystem
  Torque_sat : Saturate  UpperLimit=sat.wheel.max_torque  LowerLimit=- sat.wheel.max_torque
  Wheel Inertia : Constant  Value=sat.wheel.max_sigma/sat.wheel.max_speed
  Omega_C (scalar) : Outport
  P_w : Outport  Port=2
  wires:
  Divide/1 -> Discrete-Time Integrator/1  "dw/dt"
  Discrete-Time Integrator/1 -> Saturation_speed/1
  Mc (scalar)/1 -> Torque_sat/1
  Torque_sat/1 -> Subsystem/1(Torque (scal)), Divide/1  "Torque (scal)"
  Wheel Inertia/1 -> Subsystem/3(J_wheel), Divide/2
  Saturation_speed/1 -> Subsystem/2(omega_wheel), Omega_C (scalar)/1
  Subsystem/1(P_wheel) -> P_w/1

== system Control_v4_desat0/Attitude Controller/PID (nominal command)/RW2 ==
  note: Entrées:
      | - Moment de commande (déjà projeté sur l'axe de la roue...)
      | Sorties:
      | - Omega de commande à appliquer
  Mc (scalar) : Inport
  Discrete-Time Integrator : DiscreteIntegrator  IntegratorMethod=Integration: Trapezoidal  SampleTime=-1  ICPrevOutput=DiscIntNeverNeededParam  ICPrevScaledInput=DiscIntNeverNeededParam
  Divide : Product  Inputs=*/
  Saturation_speed : Saturate  UpperLimit=sat.wheel.max_speed  LowerLimit=- sat.wheel.max_speed
  Subsystem : Subsystem
  Torque_sat : Saturate  UpperLimit=sat.wheel.max_torque  LowerLimit=- sat.wheel.max_torque
  Wheel Inertia : Constant  Value=sat.wheel.max_sigma/sat.wheel.max_speed
  Omega_C (scalar) : Outport
  P_w : Outport  Port=2
  wires:
  Divide/1 -> Discrete-Time Integrator/1  "dw/dt"
  Discrete-Time Integrator/1 -> Saturation_speed/1
  Mc (scalar)/1 -> Torque_sat/1
  Wheel Inertia/1 -> Subsystem/3(J_wheel), Divide/2
  Torque_sat/1 -> Subsystem/1(Torque (scal)), Divide/1  "Torque (scal)"
  Saturation_speed/1 -> Subsystem/2(omega_wheel), Omega_C (scalar)/1
  Subsystem/1(P_wheel) -> P_w/1

== system Control_v4_desat0/Attitude Controller/PID (nominal command)/RW3 ==
  note: Entrées:
      | - Moment de commande (déjà projeté sur l'axe de la roue...)
      | Sorties:
      | - Omega de commande à appliquer
  Mc (scalar) : Inport
  Discrete-Time Integrator : DiscreteIntegrator  IntegratorMethod=Integration: Trapezoidal  SampleTime=-1  ICPrevOutput=DiscIntNeverNeededParam  ICPrevScaledInput=DiscIntNeverNeededParam
  Divide : Product  Inputs=*/
  Saturation_speed : Saturate  UpperLimit=sat.wheel.max_speed  LowerLimit=- sat.wheel.max_speed
  Subsystem : Subsystem
  Torque_sat : Saturate  UpperLimit=sat.wheel.max_torque  LowerLimit=- sat.wheel.max_torque
  Wheel Inertia : Constant  Value=sat.wheel.max_sigma/sat.wheel.max_speed
  Omega_C (scalar) : Outport
  P_w : Outport  Port=2
  wires:
  Divide/1 -> Discrete-Time Integrator/1  "dw/dt"
  Discrete-Time Integrator/1 -> Saturation_speed/1
  Mc (scalar)/1 -> Torque_sat/1
  Wheel Inertia/1 -> Subsystem/3(J_wheel), Divide/2
  Torque_sat/1 -> Subsystem/1(Torque (scal)), Divide/1  "Torque (scal)"
  Saturation_speed/1 -> Subsystem/2(omega_wheel), Omega_C (scalar)/1
  Subsystem/1(P_wheel) -> P_w/1

== system Control_v4_desat0/Attitude Controller/PID (nominal command)/RW4  ==
  note: Entrées:
      | - Moment de commande (déjà projeté sur l'axe de la roue...)
      | Sorties:
      | - Omega de commande à appliquer
  Mc (scalar) : Inport
  Discrete-Time Integrator : DiscreteIntegrator  IntegratorMethod=Integration: Trapezoidal  SampleTime=-1  ICPrevOutput=DiscIntNeverNeededParam  ICPrevScaledInput=DiscIntNeverNeededParam
  Divide : Product  Inputs=*/
  Saturation_speed : Saturate  UpperLimit=sat.wheel.max_speed  LowerLimit=- sat.wheel.max_speed
  Subsystem : Subsystem
  Torque_sat : Saturate  UpperLimit=sat.wheel.max_torque  LowerLimit=- sat.wheel.max_torque
  Wheel Inertia : Constant  Value=sat.wheel.max_sigma/sat.wheel.max_speed
  Omega_C (scalar) : Outport
  P_w : Outport  Port=2
  wires:
  Divide/1 -> Discrete-Time Integrator/1  "dw/dt"
  Discrete-Time Integrator/1 -> Saturation_speed/1
  Mc (scalar)/1 -> Torque_sat/1
  Wheel Inertia/1 -> Subsystem/3(J_wheel), Divide/2
  Torque_sat/1 -> Subsystem/1(Torque (scal)), Divide/1  "Torque (scal)"
  Saturation_speed/1 -> Subsystem/2(omega_wheel), Omega_C (scalar)/1
  Subsystem/1(P_wheel) -> P_w/1

== system Control_v4_desat0/Attitude Controller/Reaction Wheels Speed Command/Switch Case Action Subsystem3 ==
  In1 : Inport
  Action Port : ActionPort  ActionPortLabel=if(u1 > 0)
  Out1 : Outport  VectorParamsAs1DForOutWhenUnconnected=off
  wires:
  In1/1 -> Out1/1

== system Control_v4_desat0/Attitude Controller/Reaction Wheels Speed Command/Switch Case Action Subsystem4 ==
  In1 : Inport
  Action Port : ActionPort  ActionPortLabel=else
  Out1 : Outport  VectorParamsAs1DForOutWhenUnconnected=off
  wires:
  In1/1 -> Out1/1

== system Control_v4_desat0/Disturbance Torques/Aerodynamic Model/Calculate - Az & El Angle ==
  attitude : Inport
  Wind unit ECI : Inport  Port=2
  Atan2 : Trigonometry  Operator=atan2
  Constant1 : Constant  Value=2*pi
  Demux : Demux  Outputs=3
  Rotation : Product  Multiplication=Matrix(*)  RndMeth=Zero
  Sum : Sum  Inputs=|++
  Switch : Switch
  Trigonometric Function2 : Trigonometry  Operator=asin
  El : Outport
  Az : Outport  Port=2
  wires:
  attitude/1 -> Rotation/1  "ECI to BRF"
  Wind unit ECI/1 -> Rotation/2
  Rotation/1 -> Demux/1  "wind BRF"
  Demux/3 -> Trigonometric Function2/1
  Trigonometric Function2/1 -> El/1  "Elevation"
  Demux/1 -> Atan2/2
  Demux/2 -> Atan2/1
  Atan2/1 -> Switch/1, Switch/2, Sum/2
  Switch/1 -> Az/1
  Constant1/1 -> Sum/1
  Sum/1 -> Switch/3

== system Control_v4_desat0/Disturbance Torques/Aerodynamic Model/Get Density ==
  note: Altitude (distance to center of earth)
  <XYZ_ECI> : Inport
  DOY : Inport  Port=2
  "DCM_i2e " : Inport  Port=3
  Demux1 : Demux  Outputs=3
  Dot Product - magnitude squared : DotProduct  InputSameDT=on  OutDataTypeStr=Inherit: Inherit via internal rule
  ECI To LLA : MATLAB Function  TreatAsAtomicUnit=on
  Lookup - Air density : Lookup  InputValues=IonSataero.alt_range*1000 + 6378100  Table=IonSataero.av_density_vs_alt
  MATLAB Function2 : MATLAB Function  TreatAsAtomicUnit=on
  Mux2 : Mux  Inputs=3
  NRLMSISE-00 Atmosphere Model : aerolibatmos2/NRLMSISE-00 Atmosphere Model  units=Metric (MKS)  lst_input=off  flux_ap_input=off  flags_input=Internal  flags=ones(1,23)  oxygen_in=on  action=Warning
      settings: SourceProductBaseCode=AE
  Product : Product  Multiplication=Matrix(*)
  Reshape : Reshape  OutputDimensionality=Row vector (2-D)
  Scope : Scope  NumInputPorts=2
  Terminator : Terminator
  sqrt : Math  Operator=sqrt  SignedPower=on  SaturateOnIntegerOverflow=on
  Density Lookup table : Outport
  Density NRLMSISE : Outport  Port=2
  wires:
  Dot Product - magnitude squared/1 -> sqrt/1
  Lookup - Air density/1 -> Scope/1, Density Lookup table/1  "Density Lookup"
  sqrt/1 -> Lookup - Air density/1
  DOY/1 -> Demux1/1
  Demux1/1 -> NRLMSISE-00 Atmosphere Model/2
  Demux1/2 -> NRLMSISE-00 Atmosphere Model/3
  NRLMSISE-00 Atmosphere Model/2 -> MATLAB Function2/1(u)
  Demux1/3 -> NRLMSISE-00 Atmosphere Model/4
  Mux2/1 -> NRLMSISE-00 Atmosphere Model/1
  NRLMSISE-00 Atmosphere Model/1 -> Terminator/1
  MATLAB Function2/1(y) -> Scope/2, Density NRLMSISE/1  "Density NRLMSISE"
  Reshape/1 -> Product/1
  "DCM_i2e "/1 -> Product/2  "DCM_i2e"
  <XYZ_ECI>/1 -> Reshape/1, Dot Product - magnitude squared/1, Dot Product - magnitude squared/2
  Product/1 -> ECI To LLA/1(X_ECEF)
  ECI To LLA/2(lat) -> Mux2/1
  ECI To LLA/3(long) -> Mux2/2
  ECI To LLA/1(h) -> Mux2/3

== system Control_v4_desat0/IGRF Computation block/Obtain B_ECI/Dipole Subsystem ==
  In1 : Inport
  Action Port : ActionPort  ActionPortLabel=else
  Bus Selector1 : BusSelector  OutputSignals=h,lat,long,DCM_i2e
  Dipole Model : Subsystem  AncestorBlock=DipoleModel/Dipole Model
  "B_ECI " : Outport  VectorParamsAs1DForOutWhenUnconnected=off
  wires:
  In1/1 -> Bus Selector1/1
  Bus Selector1/1 -> Dipole Model/1(h)  "<h>"
  Bus Selector1/2 -> Dipole Model/2("lat ")  "<lat>"
  Bus Selector1/3 -> Dipole Model/3(long)  "<long>"
  Bus Selector1/4 -> Dipole Model/4(ECI2ECEF_DCM)  "<DCM_i2e>"
  Dipole Model/1("B_ECI ") -> "B_ECI "/1

== system Control_v4_desat0/IGRF Computation block/Obtain B_ECI/IGRF Subsystem ==
  In1 : Inport
  Action Port : ActionPort  ActionPortLabel=if(u1 > 0)
  Bus Selector : BusSelector  OutputSignals=DCM_i2e,h,lat,long,time_UTC
  International Geomagnetic Reference Field 12 : aerolibobsolete/International Geomagnetic Reference Field 12  units=Metric (MKS)  time_in=on  month=January  day=1  year=2020  action=None  sv_out=on
      settings: SourceProductBaseCode=AE
  Mux : Mux  Inputs=3
  NED to ECEF : MATLABFcn  MATLABFcn=NED2ecef  OutputDimensions=[3;1]  Output1D=off
  Permute Dimensions : PermuteDimensions
  Product : Product  Multiplication=Matrix(*)
  T to nT : Gain  Gain=1E-9
  Terminator{1..9} (9 alike) : Terminator
  Out1 : Outport  VectorParamsAs1DForOutWhenUnconnected=off
  wires:
  In1/1 -> Bus Selector/1
  Bus Selector/2 -> International Geomagnetic Reference Field 12/1  "<h>"
  T to nT/1 -> Out1/1
  Bus Selector/5 -> International Geomagnetic Reference Field 12/4  "<time_UTC>"
  Bus Selector/4 -> Mux/3, International Geomagnetic Reference Field 12/3  "<long>"
  Bus Selector/3 -> Mux/2, International Geomagnetic Reference Field 12/2  "<lat>"
  International Geomagnetic Reference Field 12/2 -> Terminator1/1
  International Geomagnetic Reference Field 12/10 -> Terminator9/1
  International Geomagnetic Reference Field 12/4 -> Terminator3/1
  International Geomagnetic Reference Field 12/5 -> Terminator4/1
  International Geomagnetic Reference Field 12/3 -> Terminator2/1
  International Geomagnetic Reference Field 12/1 -> Mux/1
  International Geomagnetic Reference Field 12/6 -> Terminator5/1
  International Geomagnetic Reference Field 12/8 -> Terminator7/1
  International Geomagnetic Reference Field 12/7 -> Terminator6/1
  International Geomagnetic Reference Field 12/9 -> Terminator8/1
  Bus Selector/1 -> Permute Dimensions/1  "<DCM_i2e>"
  Permute Dimensions/1 -> Product/1
  Product/1 -> T to nT/1
  Mux/1 -> NED to ECEF/1
  NED to ECEF/1 -> Product/2

== system Control_v4_desat0/Physical Model/6DOF in ECI frame/Compute Q_ECI ==
  note: https://arxiv.org/pdf/0811.2889.pdf
      | $ω = 2q^*\frac{dq}{dt}$ (13)
      |
      | $\frac{dq}{dt} = \frac{1}{2} q * ω$ (14)
  <Q_ECI> : Inport
  Omega_body : Inport  Port=2
  Gain : Gain  Gain=1/2
  Ground : Ground
  Integrator_quat : Integrator  InitialCondition=[1 0 0 0]
  Mux : Mux  Inputs=2
  Quaternion Multiplication : aerolibutil/Quaternion Multiplication
  Quaternion Normalize : sharedutil/Quaternion Normalize  aMode=aMode
      settings: SourceProductBaseCode=AE,PW,MT,UV,VE,VP
  Q_ECI : Outport  VectorParamsAs1DForOutWhenUnconnected=off
  wires:
  Quaternion Multiplication/1 -> Gain/1
  Omega_body/1 -> Mux/2
  Ground/1 -> Mux/1
  Mux/1 -> Quaternion Multiplication/2
  <Q_ECI>/1 -> Quaternion Multiplication/1
  Integrator_quat/1 -> Quaternion Normalize/1
  Gain/1 -> Integrator_quat/1
  Quaternion Normalize/1 -> Q_ECI/1  "Q_ECI"

== system Control_v4_desat0/Physical Model/Magnetorquer physics/Magnétocoupleur 1 ==
  note: les grounds représentant les limites en
      |  moment magnétique du magnétocoupleur (lié à l'intensité)
      | A définir
  m_in (scalar) : Inport
  Constant1 : Constant  Value=sat.mag_t.max_mm1
  Constant2 : Constant  Value=- sat.mag_t.max_mm1
  Constant6 : Constant  Value=sat.mag_t.axe1
  Product : Product
  Saturation Dynamic : simulink/Discontinuities/Saturation Dynamic  OutMin=[]  OutMax=[]  OutDataTypeStr=Inherit: Same as second input  OutDataType=fixdt(1, 16)  OutScaling=2^-10  DoSatur=off
  m_out (vect) : Outport  VectorParamsAs1DForOutWhenUnconnected=off
  wires:
  m_in (scalar)/1 -> Saturation Dynamic/2
  Constant2/1 -> Saturation Dynamic/3
  Constant1/1 -> Saturation Dynamic/1
  Saturation Dynamic/1 -> Product/1
  Product/1 -> m_out (vect)/1
  Constant6/1 -> Product/2

== system Control_v4_desat0/Physical Model/Magnetorquer physics/Magnétocoupleur 2 ==
  note: les grounds représentant les limites en
      |  moment magnétique du magnétocoupleur (lié à l'intensité)
      | A définir
  m_in (scalar) : Inport
  Constant : Constant  Value=- sat.mag_t.max_mm2
  Constant1 : Constant  Value=sat.mag_t.max_mm2
  Constant6 : Constant  Value=sat.mag_t.axe2
  Product : Product
  Saturation Dynamic : simulink/Discontinuities/Saturation Dynamic  OutMin=[]  OutMax=[]  OutDataTypeStr=Inherit: Same as second input  OutDataType=fixdt(1, 16)  OutScaling=2^-10  DoSatur=off
  m_out (vect) : Outport  VectorParamsAs1DForOutWhenUnconnected=off
  wires:
  m_in (scalar)/1 -> Saturation Dynamic/2
  Constant/1 -> Saturation Dynamic/3
  Constant1/1 -> Saturation Dynamic/1
  Product/1 -> m_out (vect)/1
  Constant6/1 -> Product/2
  Saturation Dynamic/1 -> Product/1

== system Control_v4_desat0/Physical Model/Magnetorquer physics/Magnétocoupleur 3 ==
  note: les grounds représentant les limites en
      |  moment magnétique du magnétocoupleur (lié à l'intensité)
      | A définir
  m_in (scalar) : Inport
  Constant1 : Constant  Value=sat.mag_t.max_mm3
  Constant2 : Constant  Value=- sat.mag_t.max_mm3
  Constant6 : Constant  Value=sat.mag_t.axe3
  Product : Product
  Saturation Dynamic : simulink/Discontinuities/Saturation Dynamic  OutMin=[]  OutMax=[]  OutDataTypeStr=Inherit: Same as second input  OutDataType=fixdt(1, 16)  OutScaling=2^-10  DoSatur=off
  m_out (vect) : Outport  VectorParamsAs1DForOutWhenUnconnected=off
  wires:
  m_in (scalar)/1 -> Saturation Dynamic/2
  Constant2/1 -> Saturation Dynamic/3
  Constant1/1 -> Saturation Dynamic/1
  Product/1 -> m_out (vect)/1
  Constant6/1 -> Product/2
  Saturation Dynamic/1 -> Product/1

== system Control_v4_desat0/Physical Model/Thruster/If Action Subsystem ==
  In1 : Inport
  Action Port : ActionPort  ActionPortLabel=if(u1)
  Out1 : Outport
  wires:
  In1/1 -> Out1/1

== system Control_v4_desat0/Physical Model/Thruster/If Action Subsystem1 ==
  In1 : Inport
  Action Port : ActionPort  ActionPortLabel=else
  Out1 : Outport
  wires:
  In1/1 -> Out1/1

== system Control_v4_desat0/Attitude Controller/PID (nominal command)/Command Magnetic moments computation/Global magnetic moment computation ==
  In1 : Inport  OutDataTypeStr=double
  In2 : Inport  Port=2
  In3 : Inport  Port=3
  In4 : Inport  Port=4
  Dot Product : DotProduct  InputSameDT=on  OutDataTypeStr=Inherit: Inherit via internal rule
  Dot Product1 : DotProduct  InputSameDT=on  OutDataTypeStr=Inherit: Inherit via internal rule
  Dot Product2 : DotProduct  InputSameDT=on  OutDataTypeStr=Inherit: Inherit via internal rule
  magnetic moment 1 (scalar) : Outport
  magnetic moment 2 (scalar) : Outport  Port=2
  magnetic moment 3 (scalar) : Outport  Port=3
  wires:
  In1/1 -> Dot Product2/1, Dot Product1/1, Dot Product/1
  In2/1 -> Dot Product/2
  In3/1 -> Dot Product1/2
  In4/1 -> Dot Product2/2
  Dot Product/1 -> magnetic moment 1 (scalar)/1
  Dot Product1/1 -> magnetic moment 2 (scalar)/1
  Dot Product2/1 -> magnetic moment 3 (scalar)/1

== system Control_v4_desat0/Attitude Controller/PID (nominal command)/RW1/Subsystem ==
  Torque (scal) : Inport
  omega_wheel : Inport  Port=2
  J_wheel : Inport  Port=3
  Constant : Constant  Value=0.47
  Dot Product : DotProduct  InputSameDT=on  OutDataTypeStr=Inherit: Inherit via internal rule
  Dot Product1 : DotProduct  InputSameDT=on  OutDataTypeStr=Inherit: Inherit via internal rule
  Gain : Gain  Gain=1e3
  Gain1 : Gain  Gain=4.5
  Power : Math  Operator=pow  SaturateOnIntegerOverflow=on
  Product : Product
  Sqrt : Sqrt  SaturateOnIntegerOverflow=on
  Sqrt1 : Sqrt  SaturateOnIntegerOverflow=on
  Sum : Sum  Inputs=|++
  P_wheel : Outport
  wires:
  Gain/1 -> Sum/1
  Power/1 -> Gain1/1
  Constant/1 -> Power/2
  Product/1 -> Power/1
  Dot Product/1 -> Sqrt/1
  Sum/1 -> P_wheel/1
  Torque (scal)/1 -> Dot Product/2, Dot Product/1
  Sqrt/1 -> Gain/1
  Gain1/1 -> Sum/2
  J_wheel/1 -> Product/2
  omega_wheel/1 -> Dot Product1/2, Dot Product1/1
  Dot Product1/1 -> Sqrt1/1
  Sqrt1/1 -> Product/1

== system Control_v4_desat0/Attitude Controller/PID (nominal command)/RW2/Subsystem ==
  Torque (scal) : Inport
  omega_wheel : Inport  Port=2
  J_wheel : Inport  Port=3
  Constant : Constant  Value=0.47
  Dot Product : DotProduct  InputSameDT=on  OutDataTypeStr=Inherit: Inherit via internal rule
  Dot Product1 : DotProduct  InputSameDT=on  OutDataTypeStr=Inherit: Inherit via internal rule
  Gain : Gain  Gain=1e3
  Gain1 : Gain  Gain=4.5
  Power : Math  Operator=pow  SaturateOnIntegerOverflow=on
  Product : Product
  Sqrt : Sqrt  SaturateOnIntegerOverflow=on
  Sqrt1 : Sqrt  SaturateOnIntegerOverflow=on
  Sum : Sum  Inputs=|++
  P_wheel : Outport
  wires:
  Gain/1 -> Sum/1
  Power/1 -> Gain1/1
  Constant/1 -> Power/2
  Product/1 -> Power/1
  Dot Product/1 -> Sqrt/1
  Sum/1 -> P_wheel/1
  Torque (scal)/1 -> Dot Product/2, Dot Product/1
  Sqrt/1 -> Gain/1
  Gain1/1 -> Sum/2
  J_wheel/1 -> Product/2
  omega_wheel/1 -> Dot Product1/2, Dot Product1/1
  Dot Product1/1 -> Sqrt1/1
  Sqrt1/1 -> Product/1

== system Control_v4_desat0/Attitude Controller/PID (nominal command)/RW3/Subsystem ==
  Torque (scal) : Inport
  omega_wheel : Inport  Port=2
  J_wheel : Inport  Port=3
  Constant : Constant  Value=0.47
  Dot Product : DotProduct  InputSameDT=on  OutDataTypeStr=Inherit: Inherit via internal rule
  Dot Product1 : DotProduct  InputSameDT=on  OutDataTypeStr=Inherit: Inherit via internal rule
  Gain : Gain  Gain=1e3
  Gain1 : Gain  Gain=4.5
  Power : Math  Operator=pow  SaturateOnIntegerOverflow=on
  Product : Product
  Sqrt : Sqrt  SaturateOnIntegerOverflow=on
  Sqrt1 : Sqrt  SaturateOnIntegerOverflow=on
  Sum : Sum  Inputs=|++
  P_wheel : Outport
  wires:
  Gain/1 -> Sum/1
  Power/1 -> Gain1/1
  Constant/1 -> Power/2
  Product/1 -> Power/1
  Dot Product/1 -> Sqrt/1
  Sum/1 -> P_wheel/1
  Torque (scal)/1 -> Dot Product/2, Dot Product/1
  Sqrt/1 -> Gain/1
  Gain1/1 -> Sum/2
  J_wheel/1 -> Product/2
  omega_wheel/1 -> Dot Product1/2, Dot Product1/1
  Dot Product1/1 -> Sqrt1/1
  Sqrt1/1 -> Product/1

== system Control_v4_desat0/Attitude Controller/PID (nominal command)/RW4 /Subsystem ==
  Torque (scal) : Inport
  omega_wheel : Inport  Port=2
  J_wheel : Inport  Port=3
  Constant : Constant  Value=0.47
  Dot Product : DotProduct  InputSameDT=on  OutDataTypeStr=Inherit: Inherit via internal rule
  Dot Product1 : DotProduct  InputSameDT=on  OutDataTypeStr=Inherit: Inherit via internal rule
  Gain : Gain  Gain=1e3
  Gain1 : Gain  Gain=4.5
  Power : Math  Operator=pow  SaturateOnIntegerOverflow=on
  Product : Product
  Sqrt : Sqrt  SaturateOnIntegerOverflow=on
  Sqrt1 : Sqrt  SaturateOnIntegerOverflow=on
  Sum : Sum  Inputs=|++
  P_wheel : Outport
  wires:
  Gain/1 -> Sum/1
  Power/1 -> Gain1/1
  Constant/1 -> Power/2
  Product/1 -> Power/1
  Dot Product/1 -> Sqrt/1
  Sum/1 -> P_wheel/1
  Torque (scal)/1 -> Dot Product/2, Dot Product/1
  Sqrt/1 -> Gain/1
  Gain1/1 -> Sum/2
  J_wheel/1 -> Product/2
  omega_wheel/1 -> Dot Product1/2, Dot Product1/1
  Dot Product1/1 -> Sqrt1/1
  Sqrt1/1 -> Product/1

== system Control_v4_desat0/IGRF Computation block/Obtain B_ECI/Dipole Subsystem/Dipole Model ==
  h : Inport
  "lat " : Inport  Port=2
  long : Inport  Port=3
  ECI2ECEF_DCM : Inport  Port=4
  Bus Creator : BusCreator  Inputs=3
  Interpreted MATLAB Function : MATLABFcn  MATLABFcn=DipoleMod(u(1),u(2),u(3),date_IGRF,nmax)
  Permute Dimensions : PermuteDimensions
  Product : Product  Multiplication=Matrix(*)
  scaling from nT to T : Gain  Gain=1e-9
  "B_ECI " : Outport  VectorParamsAs1DForOutWhenUnconnected=off
  wires:
  Product/1 -> scaling from nT to T/1
  Permute Dimensions/1 -> Product/1
  ECI2ECEF_DCM/1 -> Permute Dimensions/1
  Bus Creator/1 -> Interpreted MATLAB Function/1
  "lat "/1 -> Bus Creator/2
  long/1 -> Bus Creator/3
  scaling from nT to T/1 -> "B_ECI "/1
  Interpreted MATLAB Function/1 -> Product/2
  h/1 -> Bus Creator/1

== matlab function Control_v4_desat0/Disturbance Torques/Aerodynamic Model/Get Density/ECI To LLA ==
  data: X_ECEF input; h output; lat output; long output
function [h, lat, long] = fcn(X_ECEF)
    h = 0;
    lat = 0;
    long = 0;
[lat, long, h] = ecef2geod(X_ECEF(1),X_ECEF(2),X_ECEF(3));
